simulink model "atan2_mag_cordic_simu_v1"  (R2020b)
settings: Solver=FixedStepAuto  StartTime=0.0  StopTime=2015  FixedStep=1  RelTol=1e-3
model workspace (MAT data in the model file):
  system_noise = 0.01
libraries: hdlsllib x52, simulink x8
settings Model: FPTShortcutValueString='{{},{''BaselineRun'',1,1,1,''BaselineRun'','''',{},''M'','''',''''},{''BaselineRun_2'',1,1,1,''BaselineRun_2'','''',{},''M'','''',''''}}'  Creator=tyson  LastModifiedBy=Ethan

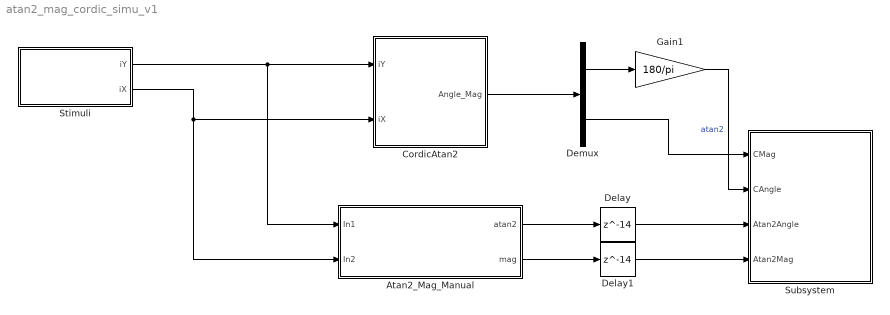
== system atan2_mag_cordic_simu_v1 ==
  Atan2_Mag_Manual : Subsystem
  CordicAtan2 : Subsystem
  Delay : Delay  DelayLength=14
  Delay1 : Delay  DelayLength=14
  Demux : Demux  Outputs=2
  Gain1 : Gain  Gain=180/pi
  Stimuli : Subsystem
  Subsystem : Subsystem
  wires:
  Atan2_Mag_Manual/2(mag) -> Delay1/1
  Atan2_Mag_Manual/1(atan2) -> Delay/1
  CordicAtan2/1(Angle_Mag) -> Demux/1
  Demux/2 -> Subsystem/1(CMag)
  Demux/1 -> Gain1/1
  Gain1/1 -> Subsystem/2(CAngle)  "atan2"
  Delay/1 -> Subsystem/3(Atan2Angle)
  Delay1/1 -> Subsystem/4(Atan2Mag)
  Stimuli/1(iY) -> CordicAtan2/1(iY), Atan2_Mag_Manual/1(In1)
  Stimuli/2(iX) -> Atan2_Mag_Manual/2(In2), CordicAtan2/2(iX)

== system atan2_mag_cordic_simu_v1/Atan2_Mag_Manual ==
  In1 : Inport
  In2 : Inport  Port=2
  Add2 : Sum
  Atan2 : Trigonometry  Operator=atan2
  Gain1 : Gain  Gain=180/pi
  Sqrt : Sqrt  SaturateOnIntegerOverflow=on
  Square : Math  Operator=square  SaturateOnIntegerOverflow=on
  Square1 : Math  Operator=square  SaturateOnIntegerOverflow=on
  atan2 : Outport
  mag : Outport  Port=2
  wires:
  In2/1 -> Square/1, Atan2/2
  Gain1/1 -> atan2/1  "atan2"
  Square/1 -> Add2/1
  Sqrt/1 -> mag/1  "mag"
  Add2/1 -> Sqrt/1
  Atan2/1 -> Gain1/1
  Square1/1 -> Add2/2
  In1/1 -> Square1/1, Atan2/1

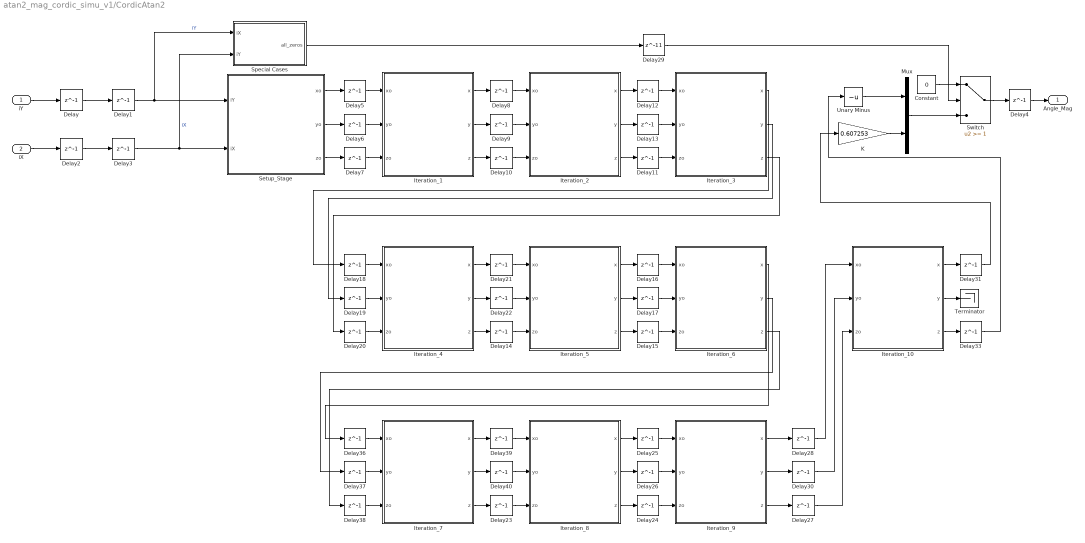
== system atan2_mag_cordic_simu_v1/CordicAtan2 ==
  iY : Inport
  iX : Inport  Port=2
  Constant : Constant  Value=0  SampleTime=-1
  Delay{,1..28,30..31,33,36..40} (37 alike) : Delay  DelayLength=1
  Delay29 : Delay  DelayLength=11
  Iteration_1 : Subsystem
  Iteration_10 : Subsystem
  Iteration_2 : Subsystem
  Iteration_3 : Subsystem
  Iteration_4 : Subsystem
  Iteration_5 : Subsystem
  Iteration_6 : Subsystem
  Iteration_7 : Subsystem
  Iteration_8 : Subsystem
  Iteration_9 : Subsystem
  K : Gain  Gain=0.607253
  Mux : Mux  Inputs=2
  Setup_Stage : Subsystem
  Special Cases : Subsystem
  Switch : Switch  Threshold=1
  Terminator : Terminator
  Unary Minus : UnaryMinus
  Angle_Mag : Outport
  wires:
  iY/1 -> Delay/1
  Delay/1 -> Delay1/1
  Delay2/1 -> Delay3/1
  iX/1 -> Delay2/1
  Constant/1 -> Switch/1
  Delay4/1 -> Angle_Mag/1
  Switch/1 -> Delay4/1
  Delay1/1 -> Setup_Stage/1(iY), Special Cases/1(iX)  "iY"
  Delay3/1 -> Special Cases/2(iY), Setup_Stage/2(iX)  "iX"
  Special Cases/1(all_zeros) -> Delay29/1
  Setup_Stage/1(xo) -> Delay5/1
  Setup_Stage/2(yo) -> Delay6/1
  Setup_Stage/3(zo) -> Delay7/1
  Delay7/1 -> Iteration_1/3(zo)
  Delay6/1 -> Iteration_1/2(yo)
  Delay5/1 -> Iteration_1/1(xo)
  Iteration_1/3(z) -> Delay10/1
  Iteration_1/1(x) -> Delay8/1
  Iteration_1/2(y) -> Delay9/1
  Delay9/1 -> Iteration_2/2(yo)
  Delay10/1 -> Iteration_2/3(zo)
  Delay8/1 -> Iteration_2/1(xo)
  Delay11/1 -> Iteration_3/3(zo)
  Delay12/1 -> Iteration_3/1(xo)
  Delay13/1 -> Iteration_3/2(yo)
  Iteration_2/2(y) -> Delay13/1
  Iteration_2/1(x) -> Delay12/1
  Iteration_2/3(z) -> Delay11/1
  Iteration_5/1(x) -> Delay16/1
  Iteration_5/2(y) -> Delay17/1
  Delay16/1 -> Iteration_6/1(xo)
  Delay17/1 -> Iteration_6/2(yo)
  Delay15/1 -> Iteration_6/3(zo)
  Iteration_5/3(z) -> Delay15/1
  Iteration_4/3(z) -> Delay14/1
  Delay14/1 -> Iteration_5/3(zo)
  Iteration_4/2(y) -> Delay22/1
  Delay21/1 -> Iteration_5/1(xo)
  Delay18/1 -> Iteration_4/1(xo)
  Delay20/1 -> Iteration_4/3(zo)
  Iteration_4/1(x) -> Delay21/1
  Delay22/1 -> Iteration_5/2(yo)
  Delay19/1 -> Iteration_4/2(yo)
  Iteration_8/1(x) -> Delay25/1
  Iteration_8/2(y) -> Delay26/1
  Delay25/1 -> Iteration_9/1(xo)
  Delay26/1 -> Iteration_9/2(yo)
  Delay24/1 -> Iteration_9/3(zo)
  Iteration_8/3(z) -> Delay24/1
  Iteration_7/3(z) -> Delay23/1
  Delay23/1 -> Iteration_8/3(zo)
  Iteration_7/2(y) -> Delay40/1
  Delay39/1 -> Iteration_8/1(xo)
  Delay36/1 -> Iteration_7/1(xo)
  Delay38/1 -> Iteration_7/3(zo)
  Iteration_7/1(x) -> Delay39/1
  Delay40/1 -> Iteration_8/2(yo)
  Delay37/1 -> Iteration_7/2(yo)
  Iteration_3/3(z) -> Delay20/1
  Iteration_3/2(y) -> Delay19/1
  Iteration_3/1(x) -> Delay18/1
  Iteration_6/3(z) -> Delay38/1
  Iteration_6/2(y) -> Delay37/1
  Iteration_6/1(x) -> Delay36/1
  Iteration_9/2(y) -> Delay30/1
  Iteration_9/1(x) -> Delay28/1
  Iteration_9/3(z) -> Delay27/1
  Mux/1 -> Switch/3
  Delay29/1 -> Switch/2
  Delay28/1 -> Iteration_10/1(xo)
  Delay30/1 -> Iteration_10/2(yo)
  Delay27/1 -> Iteration_10/3(zo)
  Iteration_10/1(x) -> Delay31/1
  Delay31/1 -> K/1
  Iteration_10/2(y) -> Terminator/1
  Iteration_10/3(z) -> Delay33/1
  Delay33/1 -> Unary Minus/1
  Unary Minus/1 -> Mux/1
  K/1 -> Mux/2

== system atan2_mag_cordic_simu_v1/Stimuli ==
  Angle Stimuli : Subsystem
  Demux : Demux  Outputs=2
  Mag Stimuli : Subsystem
  Switch : Switch  Criteria=u2 > Threshold  Threshold=1
  Switch Trigger : simulink/Sources/Repeating Sequence  rep_seq_t=[0:1:2000]  rep_seq_y=[0:(2/2000):2]
  iY : Outport
  iX : Outport  Port=2
  wires:
  Switch Trigger/1 -> Switch/2
  Demux/2 -> iX/1
  Mag Stimuli/1(Out1) -> Switch/3
  Demux/1 -> iY/1
  Angle Stimuli/1(Out1) -> Switch/1
  Switch/1 -> Demux/1

== system atan2_mag_cordic_simu_v1/Subsystem ==
  CMag : Inport
  CAngle : Inport  Port=2
  Atan2Angle : Inport  Port=3
  Atan2Mag : Inport  Port=4
  Angle Scope : Scope  NumInputPorts=2
  Atan2 : Display
  Cordic Angle : Display
  Cordic Mag : Display
  Mag : Display
  Mag Scope : Scope  NumInputPorts=2
  wires:
  CMag/1 -> Mag Scope/1, Cordic Mag/1
  CAngle/1 -> Angle Scope/1, Cordic Angle/1
  Atan2Mag/1 -> Mag Scope/2, Mag/1
  Atan2Angle/1 -> Angle Scope/2, Atan2/1

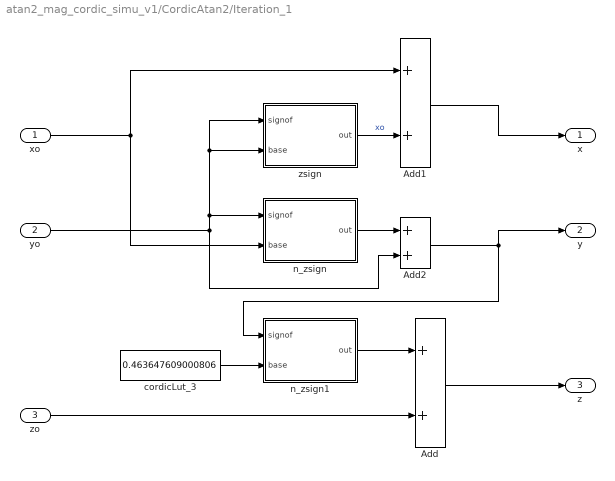
== system atan2_mag_cordic_simu_v1/CordicAtan2/Iteration_1 ==
  xo : Inport
  yo : Inport  Port=2
  zo : Inport  Port=3
  Add : Sum
  Add1 : Sum
  Add2 : Sum
  cordicLut_3 : Constant  Value=0.463647609000806  SampleTime=-1
  n_zsign : Subsystem
  n_zsign1 : Subsystem
  zsign : Subsystem
  x : Outport
  y : Outport  Port=2
  z : Outport  Port=3
  wires:
  Add/1 -> z/1
  cordicLut_3/1 -> n_zsign1/2(base)
  zo/1 -> Add/2
  n_zsign1/1(out) -> Add/1
  yo/1 -> zsign/2(base), zsign/1(signof), n_zsign/1(signof), Add2/2
  zsign/1(out) -> Add1/2  "xo"
  xo/1 -> n_zsign/2(base), Add1/1
  Add1/1 -> x/1
  n_zsign/1(out) -> Add2/1
  Add2/1 -> n_zsign1/1(signof), y/1

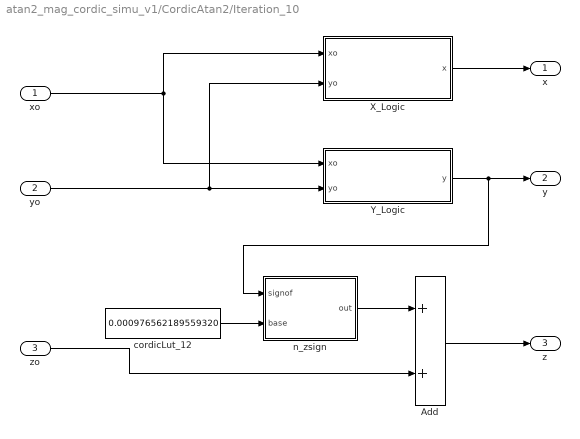
== system atan2_mag_cordic_simu_v1/CordicAtan2/Iteration_10 ==
  xo : Inport
  yo : Inport  Port=2
  zo : Inport  Port=3
  Add : Sum
  X_Logic : Subsystem
  Y_Logic : Subsystem
  cordicLut_12 : Constant  Value=0.000976562189559320  SampleTime=-1
  n_zsign : Subsystem
  x : Outport
  y : Outport  Port=2
  z : Outport  Port=3
  wires:
  Add/1 -> z/1
  cordicLut_12/1 -> n_zsign/2(base)
  zo/1 -> Add/2
  n_zsign/1(out) -> Add/1
  yo/1 -> Y_Logic/2(yo), X_Logic/2(yo)
  xo/1 -> Y_Logic/1(xo), X_Logic/1(xo)
  X_Logic/1(x) -> x/1
  Y_Logic/1(y) -> n_zsign/1(signof), y/1

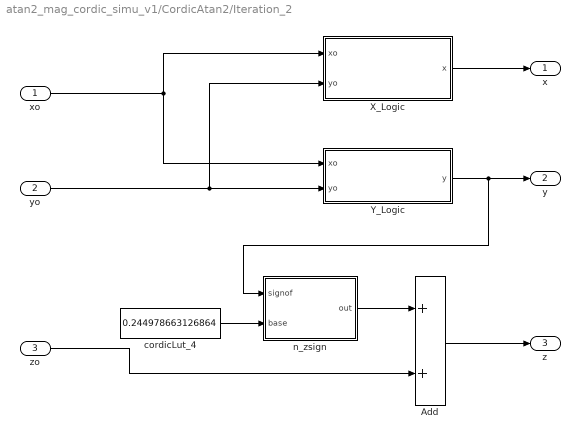
== system atan2_mag_cordic_simu_v1/CordicAtan2/Iteration_2 ==
  xo : Inport
  yo : Inport  Port=2
  zo : Inport  Port=3
  Add : Sum
  X_Logic : Subsystem
  Y_Logic : Subsystem
  cordicLut_4 : Constant  Value=0.244978663126864  SampleTime=-1
  n_zsign : Subsystem
  x : Outport
  y : Outport  Port=2
  z : Outport  Port=3
  wires:
  Add/1 -> z/1
  cordicLut_4/1 -> n_zsign/2(base)
  zo/1 -> Add/2
  n_zsign/1(out) -> Add/1
  yo/1 -> Y_Logic/2(yo), X_Logic/2(yo)
  xo/1 -> Y_Logic/1(xo), X_Logic/1(xo)
  X_Logic/1(x) -> x/1
  Y_Logic/1(y) -> n_zsign/1(signof), y/1

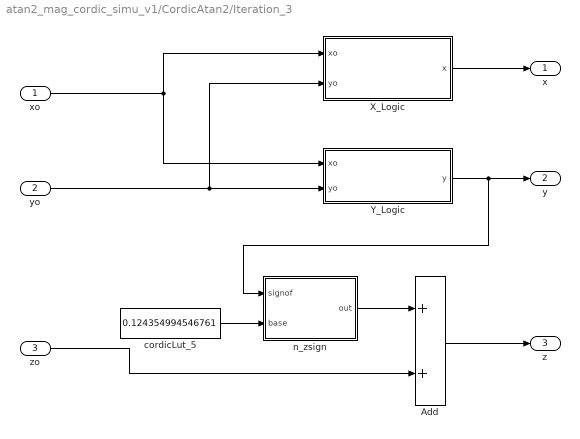
== system atan2_mag_cordic_simu_v1/CordicAtan2/Iteration_3 ==
  xo : Inport
  yo : Inport  Port=2
  zo : Inport  Port=3
  Add : Sum
  X_Logic : Subsystem
  Y_Logic : Subsystem
  cordicLut_5 : Constant  Value=0.124354994546761  SampleTime=-1
  n_zsign : Subsystem
  x : Outport
  y : Outport  Port=2
  z : Outport  Port=3
  wires:
  Add/1 -> z/1
  cordicLut_5/1 -> n_zsign/2(base)
  zo/1 -> Add/2
  n_zsign/1(out) -> Add/1
  yo/1 -> Y_Logic/2(yo), X_Logic/2(yo)
  xo/1 -> Y_Logic/1(xo), X_Logic/1(xo)
  X_Logic/1(x) -> x/1
  Y_Logic/1(y) -> n_zsign/1(signof), y/1

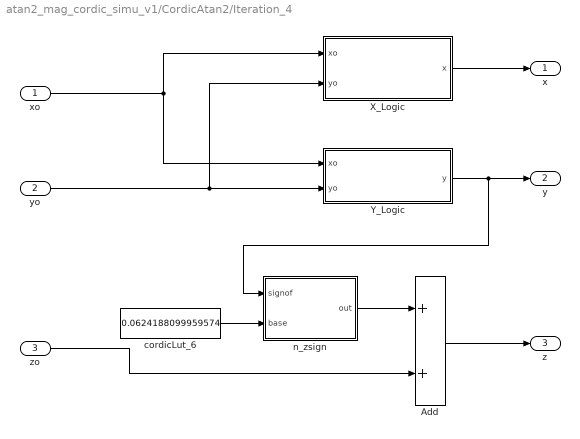
== system atan2_mag_cordic_simu_v1/CordicAtan2/Iteration_4 ==
  xo : Inport
  yo : Inport  Port=2
  zo : Inport  Port=3
  Add : Sum
  X_Logic : Subsystem
  Y_Logic : Subsystem
  cordicLut_6 : Constant  Value=0.0624188099959574  SampleTime=-1
  n_zsign : Subsystem
  x : Outport
  y : Outport  Port=2
  z : Outport  Port=3
  wires:
  Add/1 -> z/1
  cordicLut_6/1 -> n_zsign/2(base)
  zo/1 -> Add/2
  n_zsign/1(out) -> Add/1
  yo/1 -> Y_Logic/2(yo), X_Logic/2(yo)
  xo/1 -> Y_Logic/1(xo), X_Logic/1(xo)
  X_Logic/1(x) -> x/1
  Y_Logic/1(y) -> n_zsign/1(signof), y/1

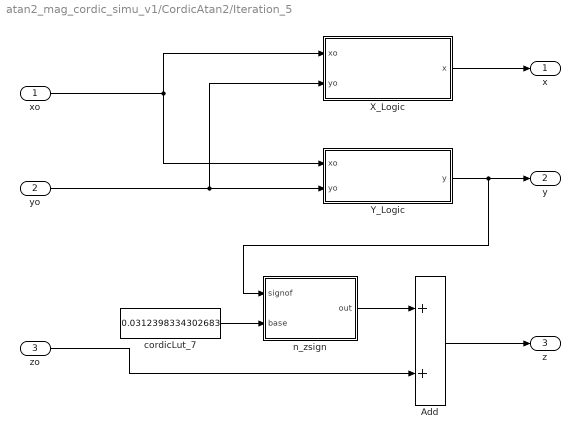
== system atan2_mag_cordic_simu_v1/CordicAtan2/Iteration_5 ==
  xo : Inport
  yo : Inport  Port=2
  zo : Inport  Port=3
  Add : Sum
  X_Logic : Subsystem
  Y_Logic : Subsystem
  cordicLut_7 : Constant  Value=0.0312398334302683  SampleTime=-1
  n_zsign : Subsystem
  x : Outport
  y : Outport  Port=2
  z : Outport  Port=3
  wires:
  Add/1 -> z/1
  cordicLut_7/1 -> n_zsign/2(base)
  zo/1 -> Add/2
  n_zsign/1(out) -> Add/1
  yo/1 -> Y_Logic/2(yo), X_Logic/2(yo)
  xo/1 -> Y_Logic/1(xo), X_Logic/1(xo)
  X_Logic/1(x) -> x/1
  Y_Logic/1(y) -> n_zsign/1(signof), y/1

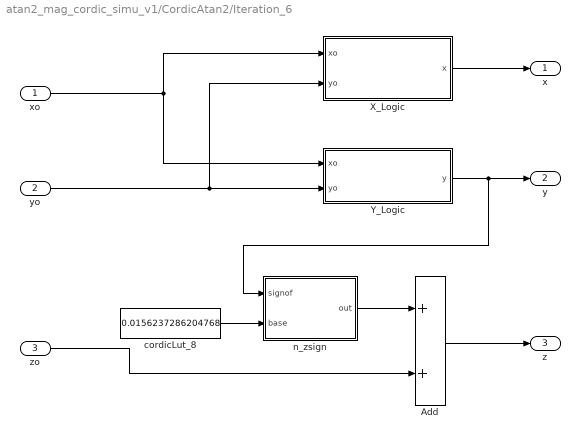
== system atan2_mag_cordic_simu_v1/CordicAtan2/Iteration_6 ==
  xo : Inport
  yo : Inport  Port=2
  zo : Inport  Port=3
  Add : Sum
  X_Logic : Subsystem
  Y_Logic : Subsystem
  cordicLut_8 : Constant  Value=0.0156237286204768  SampleTime=-1
  n_zsign : Subsystem
  x : Outport
  y : Outport  Port=2
  z : Outport  Port=3
  wires:
  Add/1 -> z/1
  cordicLut_8/1 -> n_zsign/2(base)
  zo/1 -> Add/2
  n_zsign/1(out) -> Add/1
  yo/1 -> Y_Logic/2(yo), X_Logic/2(yo)
  xo/1 -> Y_Logic/1(xo), X_Logic/1(xo)
  X_Logic/1(x) -> x/1
  Y_Logic/1(y) -> n_zsign/1(signof), y/1

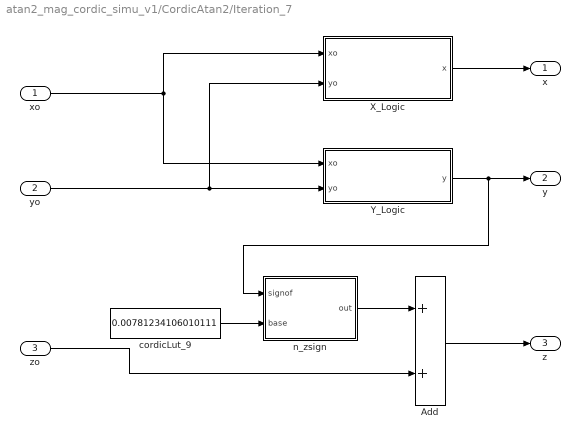
== system atan2_mag_cordic_simu_v1/CordicAtan2/Iteration_7 ==
  xo : Inport
  yo : Inport  Port=2
  zo : Inport  Port=3
  Add : Sum
  X_Logic : Subsystem
  Y_Logic : Subsystem
  cordicLut_9 : Constant  Value=0.00781234106010111  SampleTime=-1
  n_zsign : Subsystem
  x : Outport
  y : Outport  Port=2
  z : Outport  Port=3
  wires:
  Add/1 -> z/1
  cordicLut_9/1 -> n_zsign/2(base)
  zo/1 -> Add/2
  n_zsign/1(out) -> Add/1
  yo/1 -> Y_Logic/2(yo), X_Logic/2(yo)
  xo/1 -> Y_Logic/1(xo), X_Logic/1(xo)
  X_Logic/1(x) -> x/1
  Y_Logic/1(y) -> n_zsign/1(signof), y/1

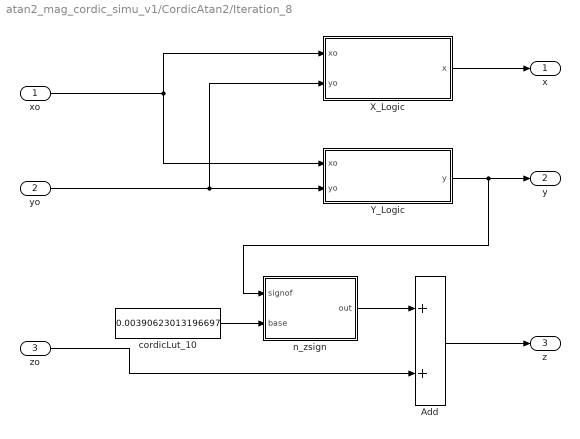
== system atan2_mag_cordic_simu_v1/CordicAtan2/Iteration_8 ==
  xo : Inport
  yo : Inport  Port=2
  zo : Inport  Port=3
  Add : Sum
  X_Logic : Subsystem
  Y_Logic : Subsystem
  cordicLut_10 : Constant  Value=0.00390623013196697  SampleTime=-1
  n_zsign : Subsystem
  x : Outport
  y : Outport  Port=2
  z : Outport  Port=3
  wires:
  Add/1 -> z/1
  cordicLut_10/1 -> n_zsign/2(base)
  zo/1 -> Add/2
  n_zsign/1(out) -> Add/1
  yo/1 -> Y_Logic/2(yo), X_Logic/2(yo)
  xo/1 -> Y_Logic/1(xo), X_Logic/1(xo)
  X_Logic/1(x) -> x/1
  Y_Logic/1(y) -> n_zsign/1(signof), y/1

== system atan2_mag_cordic_simu_v1/CordicAtan2/Iteration_9 ==
  xo : Inport
  yo : Inport  Port=2
  zo : Inport  Port=3
  Add : Sum
  X_Logic : Subsystem
  Y_Logic : Subsystem
  cordicLut_11 : Constant  Value=0.00195312251647882  SampleTime=-1
  n_zsign : Subsystem
  x : Outport
  y : Outport  Port=2
  z : Outport  Port=3
  wires:
  Add/1 -> z/1
  cordicLut_11/1 -> n_zsign/2(base)
  zo/1 -> Add/2
  n_zsign/1(out) -> Add/1
  yo/1 -> Y_Logic/2(yo), X_Logic/2(yo)
  xo/1 -> Y_Logic/1(xo), X_Logic/1(xo)
  X_Logic/1(x) -> x/1
  Y_Logic/1(y) -> n_zsign/1(signof), y/1

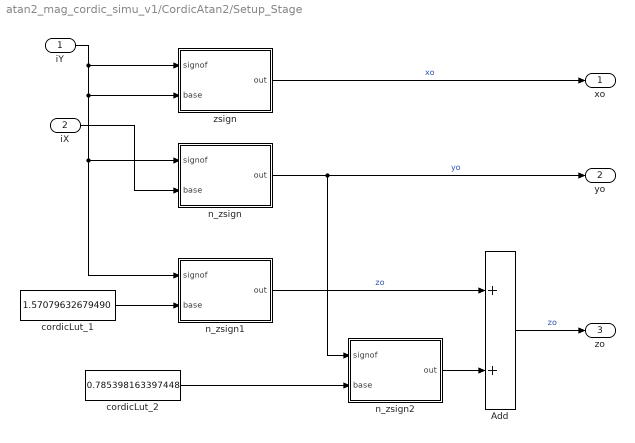
== system atan2_mag_cordic_simu_v1/CordicAtan2/Setup_Stage ==
  iY : Inport
  iX : Inport  Port=2
  Add : Sum
  cordicLut_1 : Constant  Value=1.57079632679490  SampleTime=-1
  cordicLut_2 : Constant  Value=0.785398163397448  SampleTime=-1
  n_zsign : Subsystem
  n_zsign1 : Subsystem
  n_zsign2 : Subsystem
  zsign : Subsystem
  xo : Outport
  yo : Outport  Port=2
  zo : Outport  Port=3
  wires:
  cordicLut_1/1 -> n_zsign1/2(base)
  iY/1 -> zsign/2(base), n_zsign1/1(signof), n_zsign/1(signof), zsign/1(signof)
  n_zsign/1(out) -> n_zsign2/1(signof), yo/1  "yo"
  n_zsign1/1(out) -> Add/1  "zo"
  cordicLut_2/1 -> n_zsign2/2(base)
  iX/1 -> n_zsign/2(base)
  n_zsign2/1(out) -> Add/2
  Add/1 -> zo/1  "zo"
  zsign/1(out) -> xo/1  "xo"

== system atan2_mag_cordic_simu_v1/CordicAtan2/Special Cases ==
  iX : Inport
  iY : Inport  Port=2
  Compare To Zero : simulink/Logic and Bit Operations/Compare To Zero  relop===  OutDataTypeStr=boolean
  Compare To Zero1 : simulink/Logic and Bit Operations/Compare To Zero  relop===  OutDataTypeStr=boolean
  Logical Operator : Logic  AllPortsSameDT=off  OutDataTypeStr=boolean
  all_zeros : Outport
  wires:
  Compare To Zero1/1 -> Logical Operator/2
  Logical Operator/1 -> all_zeros/1
  iY/1 -> Compare To Zero1/1
  Compare To Zero/1 -> Logical Operator/1
  iX/1 -> Compare To Zero/1

== system atan2_mag_cordic_simu_v1/Stimuli/Angle Stimuli ==
  Add : Sum
  Add1 : Sum
  Band-Limited White Noise : simulink/Sources/Band-Limited White Noise  Cov=system_noise  Ts=1  seed=[23341]
  Band-Limited White Noise1 : simulink/Sources/Band-Limited White Noise  Cov=system_noise  Ts=1  seed=[23145]
  Cos : Trigonometry  Operator=cos
  Gain : Gain  Gain=pi/180
  Mux2 : Mux  Inputs=2
  Repeating Sequence : simulink/Sources/Repeating Sequence  rep_seq_t=[0:1:1000]  rep_seq_y=[-180:(360/1000):180]
  Sin : Trigonometry
  Out1 : Outport
  wires:
  Band-Limited White Noise1/1 -> Add/2
  Gain/1 -> Sin/1, Cos/1
  Band-Limited White Noise/1 -> Add1/1
  Repeating Sequence/1 -> Gain/1
  Sin/1 -> Add/1
  Cos/1 -> Add1/2
  Mux2/1 -> Out1/1
  Add/1 -> Mux2/2
  Add1/1 -> Mux2/1

== system atan2_mag_cordic_simu_v1/Stimuli/Mag Stimuli ==
  Add1 : Sum
  Band-Limited White Noise : simulink/Sources/Band-Limited White Noise  Cov=system_noise  Ts=1  seed=[23341]
  Repeating Sequence : simulink/Sources/Repeating Sequence  rep_seq_t=[0:1:1000]  rep_seq_y=[-1:(2/1000):1]
  Out1 : Outport
  wires:
  Band-Limited White Noise/1 -> Add1/1
  Repeating Sequence/1 -> Add1/2
  Add1/1 -> Out1/1

== system atan2_mag_cordic_simu_v1/CordicAtan2/Iteration_1/n_zsign ==
  signof : Inport
  base : Inport  Port=2
  Bit Slice : hdlsllib/Logic and Bit Operations/Bit Slice  lidx=15  ridx=15
      settings: SourceProductBaseCode=SL
  Switch : Switch
  Unary Minus : UnaryMinus
  out : Outport
  wires:
  Bit Slice/1 -> Switch/2
  signof/1 -> Bit Slice/1
  Unary Minus/1 -> Switch/1
  base/1 -> Switch/3, Unary Minus/1
  Switch/1 -> out/1

== system atan2_mag_cordic_simu_v1/CordicAtan2/Iteration_1/n_zsign1 ==
  signof : Inport
  base : Inport  Port=2
  Bit Slice : hdlsllib/Logic and Bit Operations/Bit Slice  lidx=15  ridx=15
      settings: SourceProductBaseCode=SL
  Switch : Switch
  Unary Minus : UnaryMinus
  out : Outport
  wires:
  Bit Slice/1 -> Switch/2
  signof/1 -> Bit Slice/1
  Unary Minus/1 -> Switch/1
  base/1 -> Switch/3, Unary Minus/1
  Switch/1 -> out/1

== system atan2_mag_cordic_simu_v1/CordicAtan2/Iteration_1/zsign ==
  signof : Inport
  base : Inport  Port=2
  Bit Slice : hdlsllib/Logic and Bit Operations/Bit Slice  lidx=15  ridx=15
      settings: SourceProductBaseCode=SL
  Switch : Switch
  Unary Minus : UnaryMinus
  out : Outport
  wires:
  signof/1 -> Bit Slice/1
  Bit Slice/1 -> Switch/2
  base/1 -> Unary Minus/1, Switch/1
  Unary Minus/1 -> Switch/3
  Switch/1 -> out/1

== system atan2_mag_cordic_simu_v1/CordicAtan2/Iteration_10/X_Logic ==
  xo : Inport
  yo : Inport  Port=2
  Add2 : Sum
  Bit Shift : hdlsllib/Logic and Bit Operations/Bit Shift  mode=Shift Right Arithmetic  N=9
  zsign : Subsystem
  x : Outport
  wires:
  yo/1 -> Bit Shift/1, zsign/1(signof)
  Bit Shift/1 -> zsign/2(base)
  xo/1 -> Add2/1
  Add2/1 -> x/1
  zsign/1(out) -> Add2/2  "xo"

== system atan2_mag_cordic_simu_v1/CordicAtan2/Iteration_10/Y_Logic ==
  xo : Inport
  yo : Inport  Port=2
  Add1 : Sum
  Bit Shift : hdlsllib/Logic and Bit Operations/Bit Shift  mode=Shift Right Arithmetic  N=9
  n_zsign : Subsystem
  y : Outport
  wires:
  Bit Shift/1 -> n_zsign/2(base)
  n_zsign/1(out) -> Add1/2
  Add1/1 -> y/1
  xo/1 -> Bit Shift/1
  yo/1 -> n_zsign/1(signof), Add1/1

== system atan2_mag_cordic_simu_v1/CordicAtan2/Iteration_10/n_zsign ==
  signof : Inport
  base : Inport  Port=2
  Bit Slice : hdlsllib/Logic and Bit Operations/Bit Slice  lidx=15  ridx=15
      settings: SourceProductBaseCode=SL
  Switch : Switch
  Unary Minus : UnaryMinus
  out : Outport
  wires:
  Bit Slice/1 -> Switch/2
  signof/1 -> Bit Slice/1
  Unary Minus/1 -> Switch/1
  base/1 -> Switch/3, Unary Minus/1
  Switch/1 -> out/1

== system atan2_mag_cordic_simu_v1/CordicAtan2/Iteration_2/X_Logic ==
  xo : Inport
  yo : Inport  Port=2
  Add2 : Sum
  Bit Shift : hdlsllib/Logic and Bit Operations/Bit Shift  mode=Shift Right Arithmetic  N=1
  zsign : Subsystem
  x : Outport
  wires:
  yo/1 -> Bit Shift/1, zsign/1(signof)
  Bit Shift/1 -> zsign/2(base)
  xo/1 -> Add2/1
  Add2/1 -> x/1
  zsign/1(out) -> Add2/2  "xo"

== system atan2_mag_cordic_simu_v1/CordicAtan2/Iteration_2/Y_Logic ==
  xo : Inport
  yo : Inport  Port=2
  Add1 : Sum
  Bit Shift : hdlsllib/Logic and Bit Operations/Bit Shift  mode=Shift Right Arithmetic  N=1
  n_zsign : Subsystem
  y : Outport
  wires:
  Bit Shift/1 -> n_zsign/2(base)
  n_zsign/1(out) -> Add1/2
  Add1/1 -> y/1
  xo/1 -> Bit Shift/1
  yo/1 -> n_zsign/1(signof), Add1/1

== system atan2_mag_cordic_simu_v1/CordicAtan2/Iteration_2/n_zsign ==
  signof : Inport
  base : Inport  Port=2
  Bit Slice : hdlsllib/Logic and Bit Operations/Bit Slice  lidx=15  ridx=15
      settings: SourceProductBaseCode=SL
  Switch : Switch
  Unary Minus : UnaryMinus
  out : Outport
  wires:
  Bit Slice/1 -> Switch/2
  signof/1 -> Bit Slice/1
  Unary Minus/1 -> Switch/1
  base/1 -> Switch/3, Unary Minus/1
  Switch/1 -> out/1

== system atan2_mag_cordic_simu_v1/CordicAtan2/Iteration_3/X_Logic ==
  xo : Inport
  yo : Inport  Port=2
  Add2 : Sum
  Bit Shift : hdlsllib/Logic and Bit Operations/Bit Shift  mode=Shift Right Arithmetic  N=2
  zsign : Subsystem
  x : Outport
  wires:
  yo/1 -> Bit Shift/1, zsign/1(signof)
  Bit Shift/1 -> zsign/2(base)
  xo/1 -> Add2/1
  Add2/1 -> x/1
  zsign/1(out) -> Add2/2  "xo"

== system atan2_mag_cordic_simu_v1/CordicAtan2/Iteration_3/Y_Logic ==
  xo : Inport
  yo : Inport  Port=2
  Add1 : Sum
  Bit Shift : hdlsllib/Logic and Bit Operations/Bit Shift  mode=Shift Right Arithmetic  N=2
  n_zsign : Subsystem
  y : Outport
  wires:
  Bit Shift/1 -> n_zsign/2(base)
  n_zsign/1(out) -> Add1/2
  Add1/1 -> y/1
  xo/1 -> Bit Shift/1
  yo/1 -> n_zsign/1(signof), Add1/1

== system atan2_mag_cordic_simu_v1/CordicAtan2/Iteration_3/n_zsign ==
  signof : Inport
  base : Inport  Port=2
  Bit Slice : hdlsllib/Logic and Bit Operations/Bit Slice  lidx=15  ridx=15
      settings: SourceProductBaseCode=SL
  Switch : Switch
  Unary Minus : UnaryMinus
  out : Outport
  wires:
  Bit Slice/1 -> Switch/2
  signof/1 -> Bit Slice/1
  Unary Minus/1 -> Switch/1
  base/1 -> Switch/3, Unary Minus/1
  Switch/1 -> out/1

== system atan2_mag_cordic_simu_v1/CordicAtan2/Iteration_4/X_Logic ==
  xo : Inport
  yo : Inport  Port=2
  Add2 : Sum
  Bit Shift : hdlsllib/Logic and Bit Operations/Bit Shift  mode=Shift Right Arithmetic  N=3
  zsign : Subsystem
  x : Outport
  wires:
  yo/1 -> Bit Shift/1, zsign/1(signof)
  Bit Shift/1 -> zsign/2(base)
  xo/1 -> Add2/1
  Add2/1 -> x/1
  zsign/1(out) -> Add2/2  "xo"

== system atan2_mag_cordic_simu_v1/CordicAtan2/Iteration_4/Y_Logic ==
  xo : Inport
  yo : Inport  Port=2
  Add1 : Sum
  Bit Shift : hdlsllib/Logic and Bit Operations/Bit Shift  mode=Shift Right Arithmetic  N=3
  n_zsign : Subsystem
  y : Outport
  wires:
  Bit Shift/1 -> n_zsign/2(base)
  n_zsign/1(out) -> Add1/2
  Add1/1 -> y/1
  xo/1 -> Bit Shift/1
  yo/1 -> n_zsign/1(signof), Add1/1

== system atan2_mag_cordic_simu_v1/CordicAtan2/Iteration_4/n_zsign ==
  signof : Inport
  base : Inport  Port=2
  Bit Slice : hdlsllib/Logic and Bit Operations/Bit Slice  lidx=15  ridx=15
      settings: SourceProductBaseCode=SL
  Switch : Switch
  Unary Minus : UnaryMinus
  out : Outport
  wires:
  Bit Slice/1 -> Switch/2
  signof/1 -> Bit Slice/1
  Unary Minus/1 -> Switch/1
  base/1 -> Switch/3, Unary Minus/1
  Switch/1 -> out/1

== system atan2_mag_cordic_simu_v1/CordicAtan2/Iteration_5/X_Logic ==
  xo : Inport
  yo : Inport  Port=2
  Add2 : Sum
  Bit Shift : hdlsllib/Logic and Bit Operations/Bit Shift  mode=Shift Right Arithmetic  N=4
  zsign : Subsystem
  x : Outport
  wires:
  yo/1 -> Bit Shift/1, zsign/1(signof)
  Bit Shift/1 -> zsign/2(base)
  xo/1 -> Add2/1
  Add2/1 -> x/1
  zsign/1(out) -> Add2/2  "xo"

== system atan2_mag_cordic_simu_v1/CordicAtan2/Iteration_5/Y_Logic ==
  xo : Inport
  yo : Inport  Port=2
  Add1 : Sum
  Bit Shift : hdlsllib/Logic and Bit Operations/Bit Shift  mode=Shift Right Arithmetic  N=4
  n_zsign : Subsystem
  y : Outport
  wires:
  Bit Shift/1 -> n_zsign/2(base)
  n_zsign/1(out) -> Add1/2
  Add1/1 -> y/1
  xo/1 -> Bit Shift/1
  yo/1 -> n_zsign/1(signof), Add1/1

== system atan2_mag_cordic_simu_v1/CordicAtan2/Iteration_5/n_zsign ==
  signof : Inport
  base : Inport  Port=2
  Bit Slice : hdlsllib/Logic and Bit Operations/Bit Slice  lidx=15  ridx=15
      settings: SourceProductBaseCode=SL
  Switch : Switch
  Unary Minus : UnaryMinus
  out : Outport
  wires:
  Bit Slice/1 -> Switch/2
  signof/1 -> Bit Slice/1
  Unary Minus/1 -> Switch/1
  base/1 -> Switch/3, Unary Minus/1
  Switch/1 -> out/1

== system atan2_mag_cordic_simu_v1/CordicAtan2/Iteration_6/X_Logic ==
  xo : Inport
  yo : Inport  Port=2
  Add2 : Sum
  Bit Shift : hdlsllib/Logic and Bit Operations/Bit Shift  mode=Shift Right Arithmetic  N=5
  zsign : Subsystem
  x : Outport
  wires:
  yo/1 -> Bit Shift/1, zsign/1(signof)
  Bit Shift/1 -> zsign/2(base)
  xo/1 -> Add2/1
  Add2/1 -> x/1
  zsign/1(out) -> Add2/2  "xo"

== system atan2_mag_cordic_simu_v1/CordicAtan2/Iteration_6/Y_Logic ==
  xo : Inport
  yo : Inport  Port=2
  Add1 : Sum
  Bit Shift : hdlsllib/Logic and Bit Operations/Bit Shift  mode=Shift Right Arithmetic  N=5
  n_zsign : Subsystem
  y : Outport
  wires:
  Bit Shift/1 -> n_zsign/2(base)
  n_zsign/1(out) -> Add1/2
  Add1/1 -> y/1
  xo/1 -> Bit Shift/1
  yo/1 -> n_zsign/1(signof), Add1/1

== system atan2_mag_cordic_simu_v1/CordicAtan2/Iteration_6/n_zsign ==
  signof : Inport
  base : Inport  Port=2
  Bit Slice : hdlsllib/Logic and Bit Operations/Bit Slice  lidx=15  ridx=15
      settings: SourceProductBaseCode=SL
  Switch : Switch
  Unary Minus : UnaryMinus
  out : Outport
  wires:
  Bit Slice/1 -> Switch/2
  signof/1 -> Bit Slice/1
  Unary Minus/1 -> Switch/1
  base/1 -> Switch/3, Unary Minus/1
  Switch/1 -> out/1

== system atan2_mag_cordic_simu_v1/CordicAtan2/Iteration_7/X_Logic ==
  xo : Inport
  yo : Inport  Port=2
  Add2 : Sum
  Bit Shift : hdlsllib/Logic and Bit Operations/Bit Shift  mode=Shift Right Arithmetic  N=6
  zsign : Subsystem
  x : Outport
  wires:
  yo/1 -> Bit Shift/1, zsign/1(signof)
  Bit Shift/1 -> zsign/2(base)
  xo/1 -> Add2/1
  Add2/1 -> x/1
  zsign/1(out) -> Add2/2  "xo"

== system atan2_mag_cordic_simu_v1/CordicAtan2/Iteration_7/Y_Logic ==
  xo : Inport
  yo : Inport  Port=2
  Add1 : Sum
  Bit Shift : hdlsllib/Logic and Bit Operations/Bit Shift  mode=Shift Right Arithmetic  N=6
  n_zsign : Subsystem
  y : Outport
  wires:
  Bit Shift/1 -> n_zsign/2(base)
  n_zsign/1(out) -> Add1/2
  Add1/1 -> y/1
  xo/1 -> Bit Shift/1
  yo/1 -> n_zsign/1(signof), Add1/1

== system atan2_mag_cordic_simu_v1/CordicAtan2/Iteration_7/n_zsign ==
  signof : Inport
  base : Inport  Port=2
  Bit Slice : hdlsllib/Logic and Bit Operations/Bit Slice  lidx=15  ridx=15
      settings: SourceProductBaseCode=SL
  Switch : Switch
  Unary Minus : UnaryMinus
  out : Outport
  wires:
  Bit Slice/1 -> Switch/2
  signof/1 -> Bit Slice/1
  Unary Minus/1 -> Switch/1
  base/1 -> Switch/3, Unary Minus/1
  Switch/1 -> out/1

== system atan2_mag_cordic_simu_v1/CordicAtan2/Iteration_8/X_Logic ==
  xo : Inport
  yo : Inport  Port=2
  Add2 : Sum
  Bit Shift : hdlsllib/Logic and Bit Operations/Bit Shift  mode=Shift Right Arithmetic  N=7
  zsign : Subsystem
  x : Outport
  wires:
  yo/1 -> Bit Shift/1, zsign/1(signof)
  Bit Shift/1 -> zsign/2(base)
  xo/1 -> Add2/1
  Add2/1 -> x/1
  zsign/1(out) -> Add2/2  "xo"

== system atan2_mag_cordic_simu_v1/CordicAtan2/Iteration_8/Y_Logic ==
  xo : Inport
  yo : Inport  Port=2
  Add1 : Sum
  Bit Shift : hdlsllib/Logic and Bit Operations/Bit Shift  mode=Shift Right Arithmetic  N=7
  n_zsign : Subsystem
  y : Outport
  wires:
  Bit Shift/1 -> n_zsign/2(base)
  n_zsign/1(out) -> Add1/2
  Add1/1 -> y/1
  xo/1 -> Bit Shift/1
  yo/1 -> n_zsign/1(signof), Add1/1

== system atan2_mag_cordic_simu_v1/CordicAtan2/Iteration_8/n_zsign ==
  signof : Inport
  base : Inport  Port=2
  Bit Slice : hdlsllib/Logic and Bit Operations/Bit Slice  lidx=15  ridx=15
      settings: SourceProductBaseCode=SL
  Switch : Switch
  Unary Minus : UnaryMinus
  out : Outport
  wires:
  Bit Slice/1 -> Switch/2
  signof/1 -> Bit Slice/1
  Unary Minus/1 -> Switch/1
  base/1 -> Switch/3, Unary Minus/1
  Switch/1 -> out/1

== system atan2_mag_cordic_simu_v1/CordicAtan2/Iteration_9/X_Logic ==
  xo : Inport
  yo : Inport  Port=2
  Add2 : Sum
  Bit Shift : hdlsllib/Logic and Bit Operations/Bit Shift  mode=Shift Right Arithmetic  N=8
  zsign : Subsystem
  x : Outport
  wires:
  yo/1 -> Bit Shift/1, zsign/1(signof)
  Bit Shift/1 -> zsign/2(base)
  xo/1 -> Add2/1
  Add2/1 -> x/1
  zsign/1(out) -> Add2/2  "xo"

== system atan2_mag_cordic_simu_v1/CordicAtan2/Iteration_9/Y_Logic ==
  xo : Inport
  yo : Inport  Port=2
  Add1 : Sum
  Bit Shift : hdlsllib/Logic and Bit Operations/Bit Shift  mode=Shift Right Arithmetic  N=8
  n_zsign : Subsystem
  y : Outport
  wires:
  Bit Shift/1 -> n_zsign/2(base)
  n_zsign/1(out) -> Add1/2
  Add1/1 -> y/1
  xo/1 -> Bit Shift/1
  yo/1 -> n_zsign/1(signof), Add1/1

== system atan2_mag_cordic_simu_v1/CordicAtan2/Iteration_9/n_zsign ==
  signof : Inport
  base : Inport  Port=2
  Bit Slice : hdlsllib/Logic and Bit Operations/Bit Slice  lidx=15  ridx=15
      settings: SourceProductBaseCode=SL
  Switch : Switch
  Unary Minus : UnaryMinus
  out : Outport
  wires:
  Bit Slice/1 -> Switch/2
  signof/1 -> Bit Slice/1
  Unary Minus/1 -> Switch/1
  base/1 -> Switch/3, Unary Minus/1
  Switch/1 -> out/1

== system atan2_mag_cordic_simu_v1/CordicAtan2/Setup_Stage/n_zsign ==
  signof : Inport
  base : Inport  Port=2
  Bit Slice : hdlsllib/Logic and Bit Operations/Bit Slice  lidx=15  ridx=15
      settings: SourceProductBaseCode=SL
  Switch : Switch
  Unary Minus : UnaryMinus
  out : Outport
  wires:
  Bit Slice/1 -> Switch/2
  signof/1 -> Bit Slice/1
  Unary Minus/1 -> Switch/1
  base/1 -> Switch/3, Unary Minus/1
  Switch/1 -> out/1

== system atan2_mag_cordic_simu_v1/CordicAtan2/Setup_Stage/n_zsign1 ==
  signof : Inport
  base : Inport  Port=2
  Bit Slice : hdlsllib/Logic and Bit Operations/Bit Slice  lidx=15  ridx=15
      settings: SourceProductBaseCode=SL
  Switch : Switch
  Unary Minus : UnaryMinus
  out : Outport
  wires:
  Bit Slice/1 -> Switch/2
  signof/1 -> Bit Slice/1
  Unary Minus/1 -> Switch/1
  base/1 -> Switch/3, Unary Minus/1
  Switch/1 -> out/1

== system atan2_mag_cordic_simu_v1/CordicAtan2/Setup_Stage/n_zsign2 ==
  signof : Inport
  base : Inport  Port=2
  Bit Slice : hdlsllib/Logic and Bit Operations/Bit Slice  lidx=15  ridx=15
      settings: SourceProductBaseCode=SL
  Switch : Switch
  Unary Minus : UnaryMinus
  out : Outport
  wires:
  Bit Slice/1 -> Switch/2
  signof/1 -> Bit Slice/1
  Unary Minus/1 -> Switch/1
  base/1 -> Switch/3, Unary Minus/1
  Switch/1 -> out/1

== system atan2_mag_cordic_simu_v1/CordicAtan2/Setup_Stage/zsign ==
  signof : Inport
  base : Inport  Port=2
  Bit Slice : hdlsllib/Logic and Bit Operations/Bit Slice  lidx=15  ridx=15
      settings: SourceProductBaseCode=SL
  Switch : Switch
  Unary Minus : UnaryMinus
  out : Outport
  wires:
  signof/1 -> Bit Slice/1
  Bit Slice/1 -> Switch/2
  base/1 -> Unary Minus/1, Switch/1
  Unary Minus/1 -> Switch/3
  Switch/1 -> out/1

== system atan2_mag_cordic_simu_v1/CordicAtan2/Iteration_10/X_Logic/zsign ==
  signof : Inport
  base : Inport  Port=2
  Bit Slice : hdlsllib/Logic and Bit Operations/Bit Slice  lidx=15  ridx=15
      settings: SourceProductBaseCode=SL
  Switch : Switch
  Unary Minus : UnaryMinus
  out : Outport
  wires:
  signof/1 -> Bit Slice/1
  Bit Slice/1 -> Switch/2
  base/1 -> Switch/1, Unary Minus/1
  Unary Minus/1 -> Switch/3
  Switch/1 -> out/1

== system atan2_mag_cordic_simu_v1/CordicAtan2/Iteration_10/Y_Logic/n_zsign ==
  signof : Inport
  base : Inport  Port=2
  Bit Slice : hdlsllib/Logic and Bit Operations/Bit Slice  lidx=15  ridx=15
      settings: SourceProductBaseCode=SL
  Switch : Switch
  Unary Minus : UnaryMinus
  out : Outport
  wires:
  Bit Slice/1 -> Switch/2
  signof/1 -> Bit Slice/1
  Unary Minus/1 -> Switch/1
  base/1 -> Switch/3, Unary Minus/1
  Switch/1 -> out/1

== system atan2_mag_cordic_simu_v1/CordicAtan2/Iteration_2/X_Logic/zsign ==
  signof : Inport
  base : Inport  Port=2
  Bit Slice : hdlsllib/Logic and Bit Operations/Bit Slice  lidx=15  ridx=15
      settings: SourceProductBaseCode=SL
  Switch : Switch
  Unary Minus : UnaryMinus
  out : Outport
  wires:
  signof/1 -> Bit Slice/1
  Bit Slice/1 -> Switch/2
  base/1 -> Switch/1, Unary Minus/1
  Unary Minus/1 -> Switch/3
  Switch/1 -> out/1

== system atan2_mag_cordic_simu_v1/CordicAtan2/Iteration_2/Y_Logic/n_zsign ==
  signof : Inport
  base : Inport  Port=2
  Bit Slice : hdlsllib/Logic and Bit Operations/Bit Slice  lidx=15  ridx=15
      settings: SourceProductBaseCode=SL
  Switch : Switch
  Unary Minus : UnaryMinus
  out : Outport
  wires:
  Bit Slice/1 -> Switch/2
  signof/1 -> Bit Slice/1
  Unary Minus/1 -> Switch/1
  base/1 -> Switch/3, Unary Minus/1
  Switch/1 -> out/1

== system atan2_mag_cordic_simu_v1/CordicAtan2/Iteration_3/X_Logic/zsign ==
  signof : Inport
  base : Inport  Port=2
  Bit Slice : hdlsllib/Logic and Bit Operations/Bit Slice  lidx=15  ridx=15
      settings: SourceProductBaseCode=SL
  Switch : Switch
  Unary Minus : UnaryMinus
  out : Outport
  wires:
  signof/1 -> Bit Slice/1
  Bit Slice/1 -> Switch/2
  base/1 -> Switch/1, Unary Minus/1
  Unary Minus/1 -> Switch/3
  Switch/1 -> out/1

== system atan2_mag_cordic_simu_v1/CordicAtan2/Iteration_3/Y_Logic/n_zsign ==
  signof : Inport
  base : Inport  Port=2
  Bit Slice : hdlsllib/Logic and Bit Operations/Bit Slice  lidx=15  ridx=15
      settings: SourceProductBaseCode=SL
  Switch : Switch
  Unary Minus : UnaryMinus
  out : Outport
  wires:
  Bit Slice/1 -> Switch/2
  signof/1 -> Bit Slice/1
  Unary Minus/1 -> Switch/1
  base/1 -> Switch/3, Unary Minus/1
  Switch/1 -> out/1

== system atan2_mag_cordic_simu_v1/CordicAtan2/Iteration_4/X_Logic/zsign ==
  signof : Inport
  base : Inport  Port=2
  Bit Slice : hdlsllib/Logic and Bit Operations/Bit Slice  lidx=15  ridx=15
      settings: SourceProductBaseCode=SL
  Switch : Switch
  Unary Minus : UnaryMinus
  out : Outport
  wires:
  signof/1 -> Bit Slice/1
  Bit Slice/1 -> Switch/2
  base/1 -> Switch/1, Unary Minus/1
  Unary Minus/1 -> Switch/3
  Switch/1 -> out/1

== system atan2_mag_cordic_simu_v1/CordicAtan2/Iteration_4/Y_Logic/n_zsign ==
  signof : Inport
  base : Inport  Port=2
  Bit Slice : hdlsllib/Logic and Bit Operations/Bit Slice  lidx=15  ridx=15
      settings: SourceProductBaseCode=SL
  Switch : Switch
  Unary Minus : UnaryMinus
  out : Outport
  wires:
  Bit Slice/1 -> Switch/2
  signof/1 -> Bit Slice/1
  Unary Minus/1 -> Switch/1
  base/1 -> Switch/3, Unary Minus/1
  Switch/1 -> out/1

== system atan2_mag_cordic_simu_v1/CordicAtan2/Iteration_5/X_Logic/zsign ==
  signof : Inport
  base : Inport  Port=2
  Bit Slice : hdlsllib/Logic and Bit Operations/Bit Slice  lidx=15  ridx=15
      settings: SourceProductBaseCode=SL
  Switch : Switch
  Unary Minus : UnaryMinus
  out : Outport
  wires:
  signof/1 -> Bit Slice/1
  Bit Slice/1 -> Switch/2
  base/1 -> Switch/1, Unary Minus/1
  Unary Minus/1 -> Switch/3
  Switch/1 -> out/1

== system atan2_mag_cordic_simu_v1/CordicAtan2/Iteration_5/Y_Logic/n_zsign ==
  signof : Inport
  base : Inport  Port=2
  Bit Slice : hdlsllib/Logic and Bit Operations/Bit Slice  lidx=15  ridx=15
      settings: SourceProductBaseCode=SL
  Switch : Switch
  Unary Minus : UnaryMinus
  out : Outport
  wires:
  Bit Slice/1 -> Switch/2
  signof/1 -> Bit Slice/1
  Unary Minus/1 -> Switch/1
  base/1 -> Switch/3, Unary Minus/1
  Switch/1 -> out/1

== system atan2_mag_cordic_simu_v1/CordicAtan2/Iteration_6/X_Logic/zsign ==
  signof : Inport
  base : Inport  Port=2
  Bit Slice : hdlsllib/Logic and Bit Operations/Bit Slice  lidx=15  ridx=15
      settings: SourceProductBaseCode=SL
  Switch : Switch
  Unary Minus : UnaryMinus
  out : Outport
  wires:
  signof/1 -> Bit Slice/1
  Bit Slice/1 -> Switch/2
  base/1 -> Switch/1, Unary Minus/1
  Unary Minus/1 -> Switch/3
  Switch/1 -> out/1

== system atan2_mag_cordic_simu_v1/CordicAtan2/Iteration_6/Y_Logic/n_zsign ==
  signof : Inport
  base : Inport  Port=2
  Bit Slice : hdlsllib/Logic and Bit Operations/Bit Slice  lidx=15  ridx=15
      settings: SourceProductBaseCode=SL
  Switch : Switch
  Unary Minus : UnaryMinus
  out : Outport
  wires:
  Bit Slice/1 -> Switch/2
  signof/1 -> Bit Slice/1
  Unary Minus/1 -> Switch/1
  base/1 -> Switch/3, Unary Minus/1
  Switch/1 -> out/1

== system atan2_mag_cordic_simu_v1/CordicAtan2/Iteration_7/X_Logic/zsign ==
  signof : Inport
  base : Inport  Port=2
  Bit Slice : hdlsllib/Logic and Bit Operations/Bit Slice  lidx=15  ridx=15
      settings: SourceProductBaseCode=SL
  Switch : Switch
  Unary Minus : UnaryMinus
  out : Outport
  wires:
  signof/1 -> Bit Slice/1
  Bit Slice/1 -> Switch/2
  base/1 -> Switch/1, Unary Minus/1
  Unary Minus/1 -> Switch/3
  Switch/1 -> out/1

== system atan2_mag_cordic_simu_v1/CordicAtan2/Iteration_7/Y_Logic/n_zsign ==
  signof : Inport
  base : Inport  Port=2
  Bit Slice : hdlsllib/Logic and Bit Operations/Bit Slice  lidx=15  ridx=15
      settings: SourceProductBaseCode=SL
  Switch : Switch
  Unary Minus : UnaryMinus
  out : Outport
  wires:
  Bit Slice/1 -> Switch/2
  signof/1 -> Bit Slice/1
  Unary Minus/1 -> Switch/1
  base/1 -> Switch/3, Unary Minus/1
  Switch/1 -> out/1

== system atan2_mag_cordic_simu_v1/CordicAtan2/Iteration_8/X_Logic/zsign ==
  signof : Inport
  base : Inport  Port=2
  Bit Slice : hdlsllib/Logic and Bit Operations/Bit Slice  lidx=15  ridx=15
      settings: SourceProductBaseCode=SL
  Switch : Switch
  Unary Minus : UnaryMinus
  out : Outport
  wires:
  signof/1 -> Bit Slice/1
  Bit Slice/1 -> Switch/2
  base/1 -> Switch/1, Unary Minus/1
  Unary Minus/1 -> Switch/3
  Switch/1 -> out/1

== system atan2_mag_cordic_simu_v1/CordicAtan2/Iteration_8/Y_Logic/n_zsign ==
  signof : Inport
  base : Inport  Port=2
  Bit Slice : hdlsllib/Logic and Bit Operations/Bit Slice  lidx=15  ridx=15
      settings: SourceProductBaseCode=SL
  Switch : Switch
  Unary Minus : UnaryMinus
  out : Outport
  wires:
  Bit Slice/1 -> Switch/2
  signof/1 -> Bit Slice/1
  Unary Minus/1 -> Switch/1
  base/1 -> Switch/3, Unary Minus/1
  Switch/1 -> out/1

== system atan2_mag_cordic_simu_v1/CordicAtan2/Iteration_9/X_Logic/zsign ==
  signof : Inport
  base : Inport  Port=2
  Bit Slice : hdlsllib/Logic and Bit Operations/Bit Slice  lidx=15  ridx=15
      settings: SourceProductBaseCode=SL
  Switch : Switch
  Unary Minus : UnaryMinus
  out : Outport
  wires:
  signof/1 -> Bit Slice/1
  Bit Slice/1 -> Switch/2
  base/1 -> Switch/1, Unary Minus/1
  Unary Minus/1 -> Switch/3
  Switch/1 -> out/1

== system atan2_mag_cordic_simu_v1/CordicAtan2/Iteration_9/Y_Logic/n_zsign ==
  signof : Inport
  base : Inport  Port=2
  Bit Slice : hdlsllib/Logic and Bit Operations/Bit Slice  lidx=15  ridx=15
      settings: SourceProductBaseCode=SL
  Switch : Switch
  Unary Minus : UnaryMinus
  out : Outport
  wires:
  Bit Slice/1 -> Switch/2
  signof/1 -> Bit Slice/1
  Unary Minus/1 -> Switch/1
  base/1 -> Switch/3, Unary Minus/1
  Switch/1 -> out/1
